simulink model "exemple1"  (R2013a)
settings: Solver=FixedStepDiscrete  StartTime=0.0  StopTime=4  RelTol=1e-3
libraries: simulink x9, commutil2 x2, dsparch4 x2, dspsigops x2, simulink_extras x1
settings Model: Creator=sebastienroy  LastModifiedBy=sebastienroy

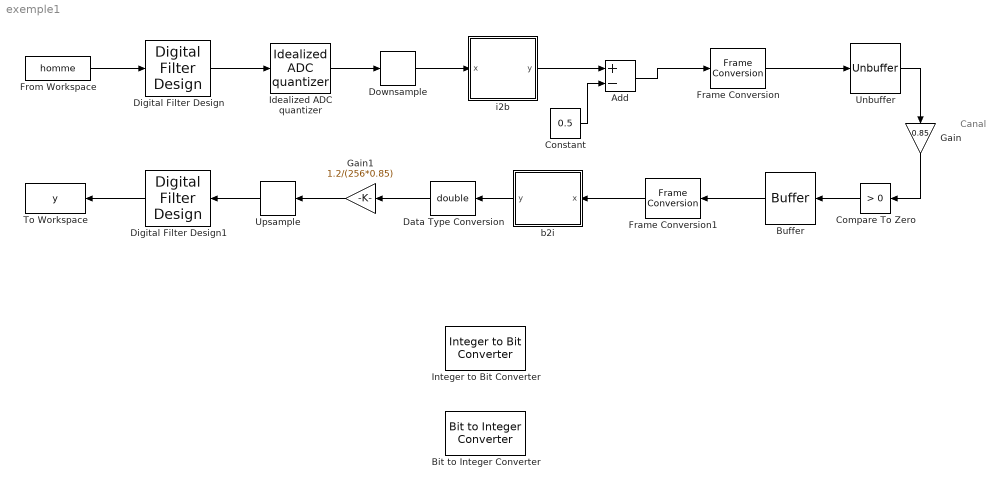
== system exemple1 ==
  note: Canal
  Add : Sum  Inputs=+-
  Bit to Integer Converter : commutil2/Bit to Integer Converter  nbits=8  bitOrder=MSB first  signedOutputValues=Signed  outDtype=Inherit via internal rule  outDtypeSigned=Inherit via internal rule
  Buffer : Buffer  N=8  TreatMby1Signals=One channel
  Compare To Zero : simulink/Logic and Bit Operations/Compare To Zero  relop=>  OutDataTypeStr=uint8
  Constant : Constant  Value=0.5
  Data Type Conversion : DataTypeConversion  OutDataTypeStr=double
  Digital Filter Design : dsparch4/Digital Filter Design  mwdsp_browser_bugfix_var=off
  Digital Filter Design1 : dsparch4/Digital Filter Design  mwdsp_browser_bugfix_var=off
  Downsample : dspsigops/Downsample  N=2  phase=0  RateOptions=Allow multirate processing  smode=Allow multirate  fmode=Maintain input frame size  ic=0
  Frame Conversion : FrameConversion
  Frame Conversion1 : FrameConversion  OutFrame=Sample-based
  From Workspace : FromWorkspace  VariableName=homme  SampleTime=6.25e-5  Interpolate=off  OutputAfterFinalValue=Setting to zero
  Gain : Gain  Gain=0.85
  Gain1 : Gain  Gain=1.2/(256*0.85)
  Idealized ADC quantizer : simulink_extras/Additional Discrete/Idealized ADC quantizer  NumberOfConverterBits=8  Vmin=-0.6  Vmax=0.6  OutputDataType=double  OutputNegativeValues=on
  Integer to Bit Converter : commutil2/Integer to Bit Converter  nbits=8  signedInputValues=Signed  bitOrder=MSB first  outDtype=Inherit via internal rule
  To Workspace : ToWorkspace  VariableName=y  SampleTime=-1
  Unbuffer : Unbuffer  SampleBasedProcessing=Same as frame based
  Upsample : dspsigops/Upsample  N=2  phase=0  RateOptions=Allow multirate processing  ic=0  mode=Unused parameter value
  b2i : Subsystem
  i2b : Subsystem
  wires:
  From Workspace/1 -> Digital Filter Design/1
  Frame Conversion/1 -> Unbuffer/1
  Idealized ADC quantizer/1 -> Downsample/1
  Downsample/1 -> i2b/1(x)
  Unbuffer/1 -> Gain/1
  Gain/1 -> Compare To Zero/1
  Buffer/1 -> Frame Conversion1/1
  Gain1/1 -> Upsample/1
  Digital Filter Design/1 -> Idealized ADC quantizer/1
  Upsample/1 -> Digital Filter Design1/1
  i2b/1(y) -> Add/1
  Add/1 -> Frame Conversion/1
  Frame Conversion1/1 -> b2i/1(x)
  Constant/1 -> Add/2
  Data Type Conversion/1 -> Gain1/1
  Compare To Zero/1 -> Buffer/1
  Digital Filter Design1/1 -> To Workspace/1
  b2i/1(y) -> Data Type Conversion/1

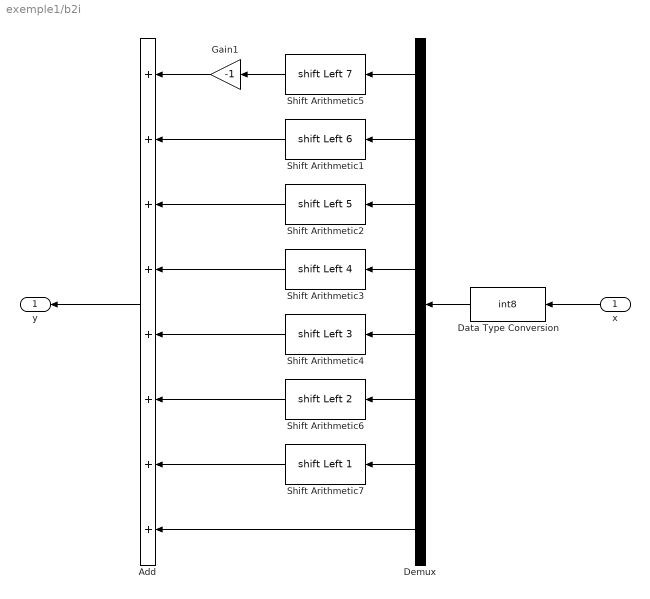
== system exemple1/b2i ==
  x : Inport
  Add : Sum  Inputs=++++++++
  Data Type Conversion : DataTypeConversion  OutDataTypeStr=int8  RndMeth=Round
  Demux : Demux  Outputs=8
  Gain1 : Gain  Gain=-1  OutDataTypeStr=int8
  Shift Arithmetic1 : ArithShift  BitShiftNumber=6  BitShiftDirection=Left
  Shift Arithmetic2 : ArithShift  BitShiftNumber=5  BitShiftDirection=Left
  Shift Arithmetic3 : ArithShift  BitShiftNumber=4  BitShiftDirection=Left
  Shift Arithmetic4 : ArithShift  BitShiftNumber=3  BitShiftDirection=Left
  Shift Arithmetic5 : ArithShift  BitShiftNumber=7  BitShiftDirection=Left
  Shift Arithmetic6 : ArithShift  BitShiftNumber=2  BitShiftDirection=Left
  Shift Arithmetic7 : ArithShift  BitShiftNumber=1  BitShiftDirection=Left
  y : Outport
  wires:
  x/1 -> Data Type Conversion/1
  Demux/1 -> Shift Arithmetic5/1
  Shift Arithmetic5/1 -> Gain1/1
  Demux/2 -> Shift Arithmetic1/1
  Demux/3 -> Shift Arithmetic2/1
  Demux/4 -> Shift Arithmetic3/1
  Demux/5 -> Shift Arithmetic4/1
  Demux/6 -> Shift Arithmetic6/1
  Demux/7 -> Shift Arithmetic7/1
  Demux/8 -> Add/8
  Shift Arithmetic7/1 -> Add/7
  Shift Arithmetic6/1 -> Add/6
  Shift Arithmetic4/1 -> Add/5
  Shift Arithmetic3/1 -> Add/4
  Shift Arithmetic2/1 -> Add/3
  Shift Arithmetic1/1 -> Add/2
  Gain1/1 -> Add/1
  Add/1 -> y/1
  Data Type Conversion/1 -> Demux/1

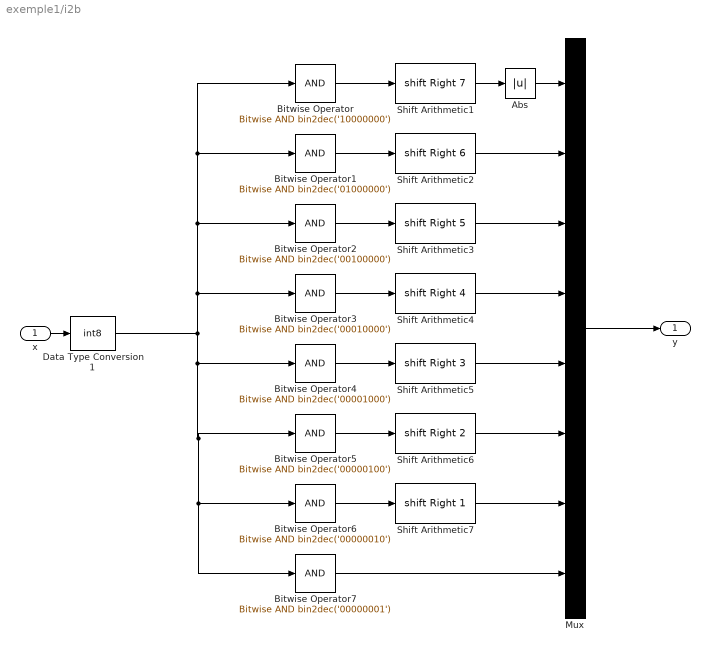
== system exemple1/i2b ==
  x : Inport
  Abs : Abs
  Bitwise Operator : simulink/Logic and Bit Operations/Bitwise Operator  logicop=AND  UseBitMask=on  BitMask=bin2dec('10000000')  BitMaskRealWorld=Stored Integer
  Bitwise Operator1 : simulink/Logic and Bit Operations/Bitwise Operator  logicop=AND  UseBitMask=on  BitMask=bin2dec('01000000')  BitMaskRealWorld=Stored Integer
  Bitwise Operator2 : simulink/Logic and Bit Operations/Bitwise Operator  logicop=AND  UseBitMask=on  BitMask=bin2dec('00100000')  BitMaskRealWorld=Stored Integer
  Bitwise Operator3 : simulink/Logic and Bit Operations/Bitwise Operator  logicop=AND  UseBitMask=on  BitMask=bin2dec('00010000')  BitMaskRealWorld=Stored Integer
  Bitwise Operator4 : simulink/Logic and Bit Operations/Bitwise Operator  logicop=AND  UseBitMask=on  BitMask=bin2dec('00001000')  BitMaskRealWorld=Stored Integer
  Bitwise Operator5 : simulink/Logic and Bit Operations/Bitwise Operator  logicop=AND  UseBitMask=on  BitMask=bin2dec('00000100')  BitMaskRealWorld=Stored Integer
  Bitwise Operator6 : simulink/Logic and Bit Operations/Bitwise Operator  logicop=AND  UseBitMask=on  BitMask=bin2dec('00000010')  BitMaskRealWorld=Stored Integer
  Bitwise Operator7 : simulink/Logic and Bit Operations/Bitwise Operator  logicop=AND  UseBitMask=on  BitMask=bin2dec('00000001')  BitMaskRealWorld=Stored Integer
  Data Type Conversion1 : DataTypeConversion  OutDataTypeStr=int8
  Mux : Mux  Inputs=8
  Shift Arithmetic1 : ArithShift  BitShiftNumber=7  BitShiftDirection=Right
  Shift Arithmetic2 : ArithShift  BitShiftNumber=6  BitShiftDirection=Right
  Shift Arithmetic3 : ArithShift  BitShiftNumber=5  BitShiftDirection=Right
  Shift Arithmetic4 : ArithShift  BitShiftNumber=4  BitShiftDirection=Right
  Shift Arithmetic5 : ArithShift  BitShiftNumber=3  BitShiftDirection=Right
  Shift Arithmetic6 : ArithShift  BitShiftNumber=2  BitShiftDirection=Right
  Shift Arithmetic7 : ArithShift  BitShiftNumber=1  BitShiftDirection=Right
  y : Outport
  wires:
  x/1 -> Data Type Conversion1/1
  Data Type Conversion1/1 -> Bitwise Operator3/1, Bitwise Operator2/1, Bitwise Operator1/1, Bitwise Operator/1, Bitwise Operator7/1, Bitwise Operator6/1, Bitwise Operator5/1, Bitwise Operator4/1
  Bitwise Operator/1 -> Shift Arithmetic1/1
  Bitwise Operator1/1 -> Shift Arithmetic2/1
  Bitwise Operator2/1 -> Shift Arithmetic3/1
  Bitwise Operator3/1 -> Shift Arithmetic4/1
  Bitwise Operator4/1 -> Shift Arithmetic5/1
  Bitwise Operator5/1 -> Shift Arithmetic6/1
  Bitwise Operator6/1 -> Shift Arithmetic7/1
  Shift Arithmetic1/1 -> Abs/1
  Shift Arithmetic2/1 -> Mux/2
  Shift Arithmetic3/1 -> Mux/3
  Shift Arithmetic4/1 -> Mux/4
  Shift Arithmetic5/1 -> Mux/5
  Shift Arithmetic6/1 -> Mux/6
  Shift Arithmetic7/1 -> Mux/7
  Bitwise Operator7/1 -> Mux/8
  Mux/1 -> y/1
  Abs/1 -> Mux/1
